simulink model "Uav_Gcs_Communication"  (R2024a)
settings: Solver=FixedStepAuto  StartTime=0.0  StopTime=inf  RelTol=1e-3
undefined symbols (not defined in the file or in its folder): Payload
libraries: uavmavlinklib x8, simulink_extras x3, instrumentlib x1
settings Model: Creator=Alireza  LastModifiedBy=mqazi
settings RTWCC: GPUComputeCapability=3.5

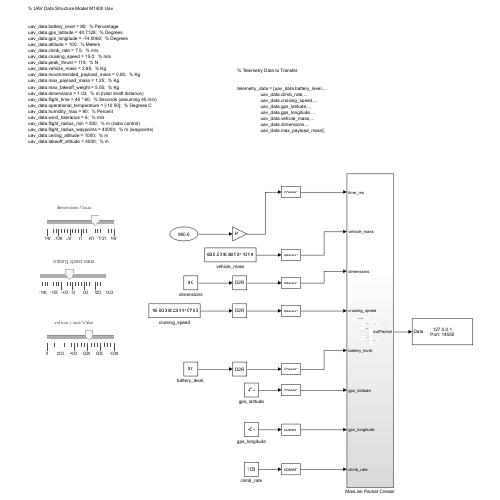
[thumbnail: Simulink's stored preview of the top-level diagram]
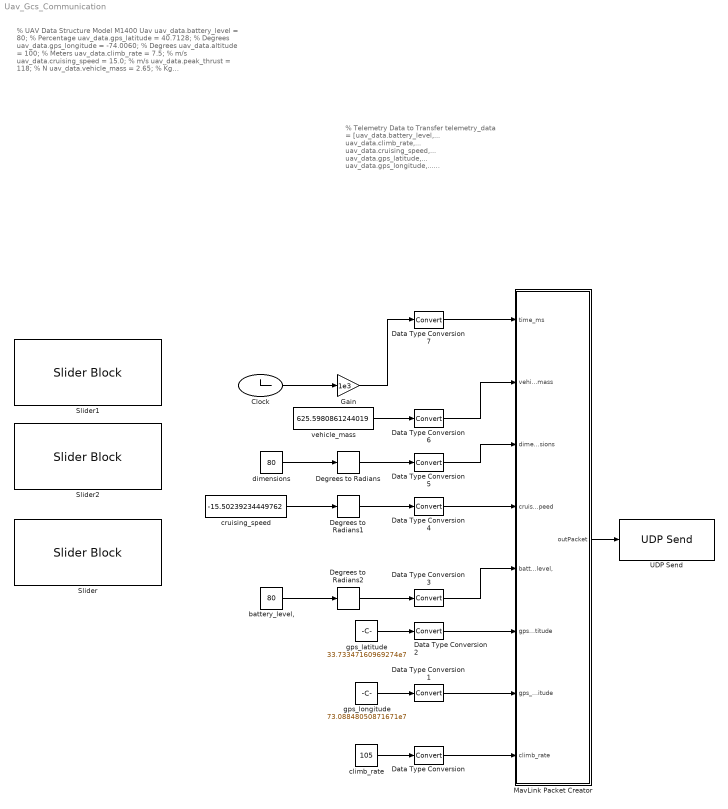
== system Uav_Gcs_Communication ==
  note: % Telemetry Data to Transfer
      |
      |
      | telemetry_data = [uav_data.battery_level,...
      |                   uav_data.climb_rate,...
      |                   uav_data.cruising_speed,...
      |                   uav_data.gps_latitude,...
      |                   uav_data.gps_longitude,...
      |                   uav_data.vehicle_mass,...
      |                   uav_data.dimensions,...
      |                   uav_data.max_payload_mass];
  note: % UAV Data Structure Model M1400 Uav
      |
      |
      | uav_data.battery_level = 80;  % Percentage
      | uav_data.gps_latitude = 40.7128;  % Degrees
      | uav_data.gps_longitude = -74.0060;  % Degrees
      | uav_data.altitude = 100;  % Meters
      | uav_data.climb_rate = 7.5;  % m/s
      | uav_data.cruising_speed = 15.0;  % m/s
      | uav_data.peak_thrust = 118;  % N
      | uav_data.vehicle_mass = 2.65;  % Kg
      | uav_data.recommended_payload_mass = 0.80;  % Kg
      | uav_data.max_payload_mass = 1.25;  % Kg
      | uav_data.max_takeoff_weight = 5.55;  % Kg
      | uav_data.dimensions = 1.03;  % m (rotor shaft distance)
      | uav_data.flight_time = 45 * 60;  % Seconds (assuming 45 min)
      | uav_data.operational_temperature = [-10 50];  % Degrees C
      | uav_data.humidity_max = 90;  % Percent
      | uav_data.wind_tolerance = 6;  % m/s
      | uav_data.flight_radius_min = 500;  % m (radio control)
      | uav_data.flight_radius_waypoints = 40000;  % m (waypoints)
      | uav_data.ceiling_altitude = 1000;  % m
      | uav_data.takeoff_altitude = 4000;  % m
  Clock : Clock
      settings: Decimation=3
  Data Type Conversion{,1..7} (8 alike) : DataTypeConversion  SaturateOnIntegerOverflow=off  RndMeth=Floor
  Degrees to Radians : simulink_extras/Transformations/Degrees to Radians
  Degrees to Radians1 : simulink_extras/Transformations/Degrees to Radians
  Degrees to Radians2 : simulink_extras/Transformations/Degrees to Radians
  Gain : Gain  Gain=1e3
  MavLink Packet Creator : Subsystem
  Slider : SliderBlock  ScaleMax=1000
  Slider1 : SliderBlock  ScaleMin=-180  ScaleMax=180
  Slider2 : SliderBlock  ScaleMin=-180  ScaleMax=180
  UDP Send : instrumentlib/UDP Send  Host=127.0.0.1  Port=14550  LocalAddress=127.0.0.1  LocalPort=-1  EnablePortSharing=off  OutputDatagramPacketSize=512  ByteOrder=big-endian  EnableBlockingMode=on  SimulateUsing=Interpreted execution
  battery_level, : Constant  Value=80  SampleTime=-1
  climb_rate : Constant  Value=105  SampleTime=-1
  cruising_speed : Constant  Value=-15.50239234449762  SampleTime=-1
  dimensions : Constant  Value=80  SampleTime=-1
  gps_latitude : Constant  Value=33.73347160969274e7  SampleTime=-1
  gps_longitude : Constant  Value=73.08848050871671e7  SampleTime=-1
  vehicle_mass : Constant  Value=625.5980861244019  SampleTime=-1
  wires:
  gps_latitude/1 -> Data Type Conversion2/1
  Clock/1 -> Gain/1
  Data Type Conversion4/1 -> MavLink Packet Creator/4(cruising_speed)
  Data Type Conversion6/1 -> MavLink Packet Creator/2(vehicle_mass)
  dimensions/1 -> Degrees to Radians/1
  battery_level,/1 -> Degrees to Radians2/1
  Degrees to Radians1/1 -> Data Type Conversion4/1
  vehicle_mass/1 -> Data Type Conversion6/1
  cruising_speed/1 -> Degrees to Radians1/1
  Gain/1 -> Data Type Conversion7/1
  Degrees to Radians/1 -> Data Type Conversion5/1
  Degrees to Radians2/1 -> Data Type Conversion3/1
  gps_longitude/1 -> Data Type Conversion1/1
  climb_rate/1 -> Data Type Conversion/1
  MavLink Packet Creator/1(outPacket) -> UDP Send/1
  Data Type Conversion7/1 -> MavLink Packet Creator/1(time_ms)
  Data Type Conversion5/1 -> MavLink Packet Creator/3(dimensions)
  Data Type Conversion1/1 -> MavLink Packet Creator/7(gps_longitude)
  Data Type Conversion3/1 -> MavLink Packet Creator/5(battery_level,)
  Data Type Conversion/1 -> MavLink Packet Creator/8(climb_rate)
  Data Type Conversion2/1 -> MavLink Packet Creator/6(gps_latitude)

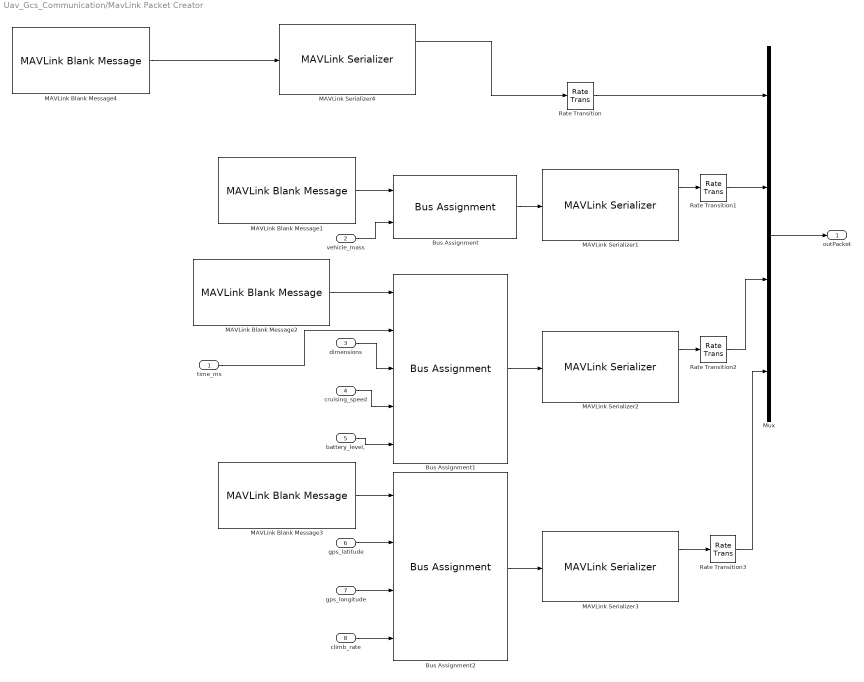
== system Uav_Gcs_Communication/MavLink Packet Creator ==
  time_ms : Inport
  vehicle_mass : Inport  Port=2
  dimensions : Inport  Port=3
  cruising_speed : Inport  Port=4
  battery_level, : Inport  Port=5
  gps_latitude : Inport  Port=6
  gps_longitude : Inport  Port=7
  climb_rate : Inport  Port=8
  Bus Assignment : BusAssignment  AssignedSignals=Payload.altitude_amsl
  Bus Assignment1 : BusAssignment  AssignedSignals=Payload.time_boot_ms,Payload.roll,Payload.pitch,Payload.yaw
  Bus Assignment2 : BusAssignment  AssignedSignals=Payload.lat,Payload.lon,Payload.alt
  MAVLink Blank Message1 : uavmavlinklib/MAVLink Blank Message  dialectSource=Select from standard MAVLink dialects  dialect=common.xml  dialectCustom=common.xml  version=2  messageType=ALTITUDE  SystemID=2  ComponentID=1  SampleTime=-1
  MAVLink Blank Message2 : uavmavlinklib/MAVLink Blank Message  dialectSource=Select from standard MAVLink dialects  dialect=common.xml  dialectCustom=common.xml  version=2  messageType=ATTITUDE  SystemID=2  ComponentID=1  SampleTime=-1
  MAVLink Blank Message3 : uavmavlinklib/MAVLink Blank Message  dialectSource=Select from standard MAVLink dialects  dialect=common.xml  dialectCustom=common.xml  version=2  messageType=GLOBAL_POSITION_INT  SystemID=2  ComponentID=1  SampleTime=-1
  MAVLink Blank Message4 : uavmavlinklib/MAVLink Blank Message  dialectSource=Select from standard MAVLink dialects  dialect=common.xml  dialectCustom=common.xml  version=2  messageType=HEARTBEAT  SystemID=2  ComponentID=1  SampleTime=-1
  MAVLink Serializer1 : uavmavlinklib/MAVLink Serializer  dialectSource=Select from standard MAVLink dialects  dialect=common.xml  dialectCustom=common.xml  version=2  messageType=ALTITUDE
  MAVLink Serializer2 : uavmavlinklib/MAVLink Serializer  dialectSource=Select from standard MAVLink dialects  dialect=common.xml  dialectCustom=common.xml  version=2  messageType=ATTITUDE
  MAVLink Serializer3 : uavmavlinklib/MAVLink Serializer  dialectSource=Select from standard MAVLink dialects  dialect=common.xml  dialectCustom=common.xml  version=2  messageType=GLOBAL_POSITION_INT
  MAVLink Serializer4 : uavmavlinklib/MAVLink Serializer  dialectSource=Select from standard MAVLink dialects  dialect=common.xml  dialectCustom=common.xml  version=2  messageType=HEARTBEAT
  Mux : Mux
  Rate Transition{,1..3} (4 alike) : RateTransition
  outPacket : Outport
  wires:
  battery_level,/1 -> Bus Assignment1/5
  dimensions/1 -> Bus Assignment1/3
  MAVLink Blank Message3/1 -> Bus Assignment2/1
  vehicle_mass/1 -> Bus Assignment/2
  MAVLink Blank Message1/1 -> Bus Assignment/1
  MAVLink Blank Message2/1 -> Bus Assignment1/1
  cruising_speed/1 -> Bus Assignment1/4
  gps_latitude/1 -> Bus Assignment2/2
  gps_longitude/1 -> Bus Assignment2/3
  climb_rate/1 -> Bus Assignment2/4
  Mux/1 -> outPacket/1
  Bus Assignment/1 -> MAVLink Serializer1/1
  Bus Assignment1/1 -> MAVLink Serializer2/1
  Bus Assignment2/1 -> MAVLink Serializer3/1
  MAVLink Serializer1/1 -> Rate Transition1/1
  MAVLink Serializer2/1 -> Rate Transition2/1
  MAVLink Serializer3/1 -> Rate Transition3/1
  Rate Transition/1 -> Mux/1
  Rate Transition1/1 -> Mux/2
  Rate Transition2/1 -> Mux/3
  Rate Transition3/1 -> Mux/4
  MAVLink Blank Message4/1 -> MAVLink Serializer4/1
  MAVLink Serializer4/1 -> Rate Transition/1
  time_ms/1 -> Bus Assignment1/2
